simulink model "WaveletDenoising1"  (R2016b)
settings: Solver=FixedStepDiscrete  StartTime=0.0  StopTime=1024  RelTol=1e-3
undefined symbols (not defined in the file or in its folder): lod, ts
libraries: dspobslib x6, dspmisc x1, dspsrcs4 x1
settings Model: ExtModeTrigMode=oneshot  ExtModeArmWhenConnect=off  ExtModeAutoUpdateStatusClock=off  Creator=The MathWorks Inc.  LastModifiedBy=admin
settings DataIOCC: SaveFormat=Array  SignalLoggingSaveFormat=ModelDataLogs  SaveOutput=off  SaveTime=off  SignalLoggingName=logsOut
settings OptimizationCC: BlockReduction=off  BooleanDataType=off  InitFltsAndDblsToZero=on  LifeSpan=inf
settings DebuggingCC: SaveWithParameterizedLinksMsg=none  UnderspecifiedInitializationDetection=Classic  MergeDetectMultiDrivingBlocksExec=none  SignalResolutionControl=TryResolveAllWithWarning  MultiTaskDSMMsg=warning  MultiTaskCondExecSysMsg=none  IntegerOverflowMsg=none  SFUnexpectedBacktrackingDiag=warning  SFNoUnconditionalDefaultTransitionDiag=warning  SFExecutionAtInitializationDiag=none  IntegerSaturationMsg=none
settings HardwareCC: ProdBitPerPointer=32  ProdBitPerSizeT=32  ProdBitPerPtrDiffT=32  ProdLargestAtomicFloat=None  ProdIntDivRoundTo=Undefined  ProdEndianess=Unspecified  ProdWordSize=32  ProdHWDeviceType=32-bit Generic  TargetUnknown=on
settings ModelReferenceCC: PropagateSignalLabelsOutOfModel=off
settings GRTTargetCC: TargetFcnLib=ansi_tfl_tmw.mat  TargetLangStandard=C89/C90 (ANSI)  CombineOutputUpdateFcns=off  GRTInterface=on
settings ConfigComp: CovMetricSettings=dw  CovHtmlReporting=on  CovSaveCumulativeToWorkspaceVar=on  CovSaveSingleToWorkspaceVar=on  CovExternalEMLEnable=off

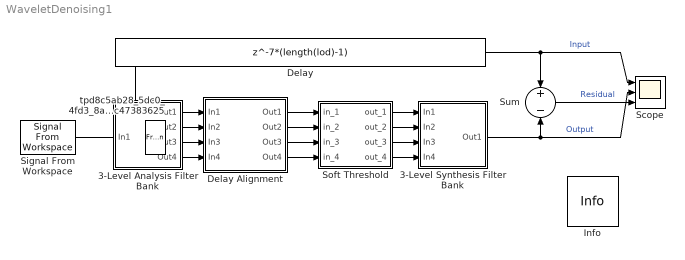
== system WaveletDenoising1 ==
  3-Level Analysis Filter Bank : Subsystem
  3-Level Synthesis Filter Bank : Subsystem
  Delay : Delay  DelayLength=7*(length(lod)-1)  InitialCondition=0  InputProcessing=Columns as channels (frame based)
  Delay Alignment : Subsystem
  Info : dspmisc/Info  SystemSampleTime=-1
  Scope : Scope  NumInputPorts=3
  Signal From Workspace : dspsrcs4/Signal From Workspace  X=signal  Ts=ts  nsamps=64  OutputAfterFinalValue=Setting to zero  ignoreOrWarnInputAndFrameLengths=off  OutputFrames=off
  Soft Threshold : Subsystem  mask(Soft Threshold){st=[2.207 2.632 1.885 1.901]}
      mask prompts: st "Vector of thresholds for each level:"
      mask help: Apply a soft threshold (deadzone transfer function) to each signal in the decomposition. First threshold applies to top-most filter bank output.
      mask init:
      | x=([-1 1 NaN 0 0 NaN -1 -.5 .5 1]+1)/2*.7+.15;
      | y=([0 0 NaN -1 1 NaN -1 0 0 1]+1)/2*.7+.05;
      mask Help: Vector of thresholds for each decomposition level.
      mask Display:
      | text(.1,.9,'Dead Zone')
      | plot(x,y)
  Sum : Sum  Inputs=+-  SaturateOnIntegerOverflow=on  InputSameDT=on  OutDataTypeStr=Inherit: Same as first input
  tpd8c5ab28_5dc0_4fd3_8a08_533c47383625 : FrameConversion  InheritSamplingMode=off
  wires:
  Soft Threshold/1(out_1) -> 3-Level Synthesis Filter Bank/1(In1)
  Soft Threshold/2(out_2) -> 3-Level Synthesis Filter Bank/2(In2)
  Soft Threshold/3(out_3) -> 3-Level Synthesis Filter Bank/3(In3)
  Soft Threshold/4(out_4) -> 3-Level Synthesis Filter Bank/4(In4)
  Delay/1 -> Sum/1, Scope/1  "Input"
  3-Level Synthesis Filter Bank/1(Out1) -> Sum/2, Scope/2  "Output"
  Sum/1 -> Scope/3  "Residual"
  3-Level Analysis Filter Bank/1(Out1) -> Delay Alignment/1(In1)
  3-Level Analysis Filter Bank/2(Out2) -> Delay Alignment/2(In2)
  3-Level Analysis Filter Bank/3(Out3) -> Delay Alignment/3(In3)
  3-Level Analysis Filter Bank/4(Out4) -> Delay Alignment/4(In4)
  Delay Alignment/1(Out1) -> Soft Threshold/1(in_1)
  Delay Alignment/2(Out2) -> Soft Threshold/2(in_2)
  Delay Alignment/3(Out3) -> Soft Threshold/3(in_3)
  Delay Alignment/4(Out4) -> Soft Threshold/4(in_4)
  Signal From Workspace/1 -> tpd8c5ab28_5dc0_4fd3_8a08_533c47383625/1
  tpd8c5ab28_5dc0_4fd3_8a08_533c47383625/1 -> 3-Level Analysis Filter Bank/1(In1), Delay/1

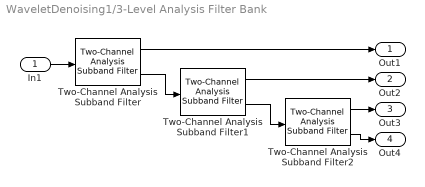
== system WaveletDenoising1/3-Level Analysis Filter Bank ==
  In1 : Inport
  Two-Channel Analysis Subband Filter : dspobslib/Two-Channel Analysis Subband Filter  lpf=lod  hpf=hid  InputProcessing=Columns as channels (frame based)  framing=Allow multirate processing  roundingMode=Floor  overflowMode=off  firstCoeffDataTypeStr=Inherit: Same word length as input  firstCoeffMin=[]  firstCoeffMax=[]  firstCoeffLastDataTypeStr=Inherit: Same word length as input  accumDataTypeStr=Inherit: Same as product output  accumLastDataTypeStr=Inherit: Same as product output  outputMin=[]  outputMax=[]
  Two-Channel Analysis Subband Filter1 : dspobslib/Two-Channel Analysis Subband Filter  lpf=lod  hpf=hid  InputProcessing=Columns as channels (frame based)  framing=Allow multirate processing  roundingMode=Floor  overflowMode=off  firstCoeffDataTypeStr=Inherit: Same word length as input  firstCoeffMin=[]  firstCoeffMax=[]  firstCoeffLastDataTypeStr=Inherit: Same word length as input  accumDataTypeStr=Inherit: Same as product output  accumLastDataTypeStr=Inherit: Same as product output  outputMin=[]  outputMax=[]
  Two-Channel Analysis Subband Filter2 : dspobslib/Two-Channel Analysis Subband Filter  lpf=lod  hpf=hid  InputProcessing=Columns as channels (frame based)  framing=Allow multirate processing  roundingMode=Floor  overflowMode=off  firstCoeffDataTypeStr=Inherit: Same word length as input  firstCoeffMin=[]  firstCoeffMax=[]  firstCoeffLastDataTypeStr=Inherit: Same word length as input  accumDataTypeStr=Inherit: Same as product output  accumLastDataTypeStr=Inherit: Same as product output  outputMin=[]  outputMax=[]
  Out1 : Outport
  Out2 : Outport  Port=2
  Out3 : Outport  Port=3
  Out4 : Outport  Port=4
  wires:
  Two-Channel Analysis Subband Filter2/2 -> Out4/1
  Two-Channel Analysis Subband Filter2/1 -> Out3/1
  Two-Channel Analysis Subband Filter1/1 -> Out2/1
  In1/1 -> Two-Channel Analysis Subband Filter/1
  Two-Channel Analysis Subband Filter/1 -> Out1/1
  Two-Channel Analysis Subband Filter1/2 -> Two-Channel Analysis Subband Filter2/1
  Two-Channel Analysis Subband Filter/2 -> Two-Channel Analysis Subband Filter1/1

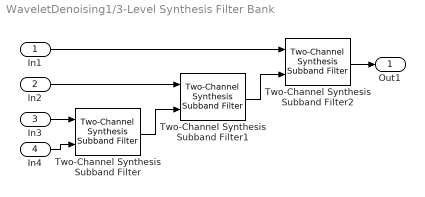
== system WaveletDenoising1/3-Level Synthesis Filter Bank ==
  In1 : Inport
  In2 : Inport  Port=2
  In3 : Inport  Port=3
  In4 : Inport  Port=4
  Two-Channel Synthesis Subband Filter : dspobslib/Two-Channel Synthesis Subband Filter  lpf=lor  hpf=hir  InputProcessing=Columns as channels (frame based)  framing=Allow multirate processing  roundingMode=Floor  overflowMode=off  firstCoeffDataTypeStr=Inherit: Same word length as input  firstCoeffMin=[]  firstCoeffMax=[]  firstCoeffLastDataTypeStr=Inherit: Same word length as input  accumDataTypeStr=Inherit: Same as product output  accumLastDataTypeStr=Inherit: Same as product output  outputDataTypeStr=Inherit: Same as accumulator  outputMin=[]  outputMax=[]  outputLastDataTypeStr=Inherit: Same as accumulator
  Two-Channel Synthesis Subband Filter1 : dspobslib/Two-Channel Synthesis Subband Filter  lpf=lor  hpf=hir  InputProcessing=Columns as channels (frame based)  framing=Allow multirate processing  roundingMode=Floor  overflowMode=off  firstCoeffDataTypeStr=Inherit: Same word length as input  firstCoeffMin=[]  firstCoeffMax=[]  firstCoeffLastDataTypeStr=Inherit: Same word length as input  accumDataTypeStr=Inherit: Same as product output  accumLastDataTypeStr=Inherit: Same as product output  outputDataTypeStr=Inherit: Same as accumulator  outputMin=[]  outputMax=[]  outputLastDataTypeStr=Inherit: Same as accumulator
  Two-Channel Synthesis Subband Filter2 : dspobslib/Two-Channel Synthesis Subband Filter  lpf=lor  hpf=hir  InputProcessing=Columns as channels (frame based)  framing=Allow multirate processing  roundingMode=Floor  overflowMode=off  firstCoeffDataTypeStr=Inherit: Same word length as input  firstCoeffMin=[]  firstCoeffMax=[]  firstCoeffLastDataTypeStr=Inherit: Same word length as input  accumDataTypeStr=Inherit: Same as product output  accumLastDataTypeStr=Inherit: Same as product output  outputDataTypeStr=Inherit: Same as accumulator  outputMin=[]  outputMax=[]  outputLastDataTypeStr=Inherit: Same as accumulator
  Out1 : Outport
  wires:
  In4/1 -> Two-Channel Synthesis Subband Filter/2
  In3/1 -> Two-Channel Synthesis Subband Filter/1
  In2/1 -> Two-Channel Synthesis Subband Filter1/1
  Two-Channel Synthesis Subband Filter2/1 -> Out1/1
  In1/1 -> Two-Channel Synthesis Subband Filter2/1
  Two-Channel Synthesis Subband Filter1/1 -> Two-Channel Synthesis Subband Filter2/2
  Two-Channel Synthesis Subband Filter/1 -> Two-Channel Synthesis Subband Filter1/2

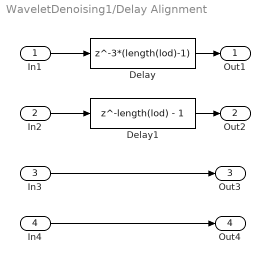
== system WaveletDenoising1/Delay Alignment ==
  In1 : Inport
  In2 : Inport  Port=2
  In3 : Inport  Port=3
  In4 : Inport  Port=4
  Delay : Delay  DelayLength=3*(length(lod)-1)  InitialCondition=0  InputProcessing=Columns as channels (frame based)
  Delay1 : Delay  DelayLength=length(lod) - 1  InitialCondition=0  InputProcessing=Columns as channels (frame based)
  Out1 : Outport
  Out2 : Outport  Port=2
  Out3 : Outport  Port=3
  Out4 : Outport  Port=4
  wires:
  In3/1 -> Out3/1
  In4/1 -> Out4/1
  In2/1 -> Delay1/1
  Delay1/1 -> Out2/1
  In1/1 -> Delay/1
  Delay/1 -> Out1/1

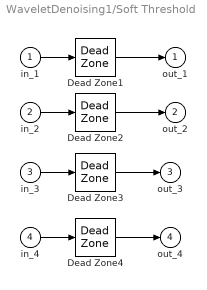
== system WaveletDenoising1/Soft Threshold ==
  in_1 : Inport
  in_2 : Inport  Port=2
  in_3 : Inport  Port=3
  in_4 : Inport  Port=4
  Dead Zone1 : DeadZone  LowerValue=-st(1)  UpperValue=st(1)  ZeroCross=off  SaturateOnIntegerOverflow=on
  Dead Zone2 : DeadZone  LowerValue=-st(2)  UpperValue=st(2)  ZeroCross=off  SaturateOnIntegerOverflow=on
  Dead Zone3 : DeadZone  LowerValue=-st(3)  UpperValue=st(3)  ZeroCross=off  SaturateOnIntegerOverflow=on
  Dead Zone4 : DeadZone  LowerValue=-st(4)  UpperValue=st(4)  ZeroCross=off  SaturateOnIntegerOverflow=on
  out_1 : Outport
  out_2 : Outport  Port=2
  out_3 : Outport  Port=3
  out_4 : Outport  Port=4
  wires:
  in_1/1 -> Dead Zone1/1
  Dead Zone1/1 -> out_1/1
  in_2/1 -> Dead Zone2/1
  Dead Zone2/1 -> out_2/1
  in_3/1 -> Dead Zone3/1
  Dead Zone3/1 -> out_3/1
  in_4/1 -> Dead Zone4/1
  Dead Zone4/1 -> out_4/1
